simulink model "PICController"  (R2022a)
settings: Solver=VariableStepAuto  StartTime=0.0  StopTime=1  RelTol=1e-3
settings Model: Creator=Jagadeesh  LastModifiedBy=Jagadeesh

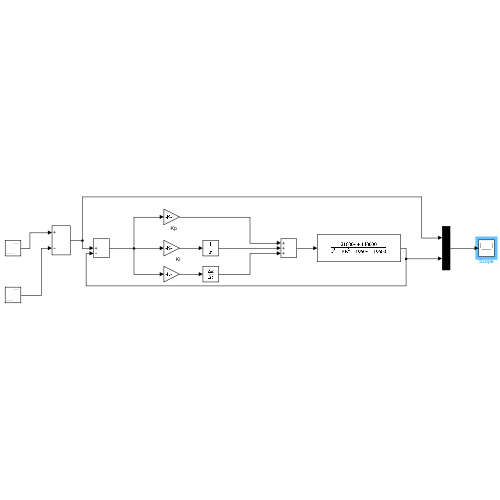
[thumbnail: Simulink's stored preview of the top-level diagram]
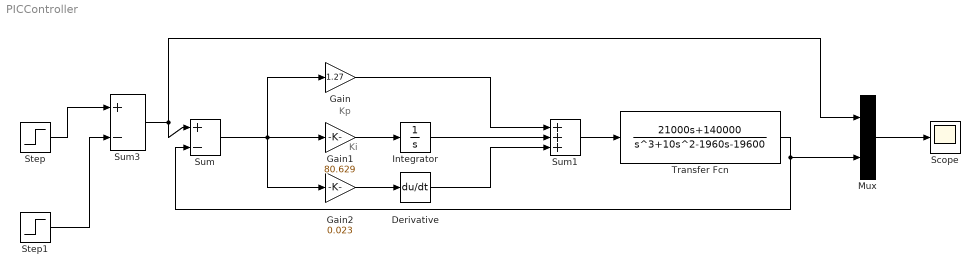
== system PICController ==
  note: Ki
  note: Kp
  Derivative : Derivative
  Gain : Gain  Gain=1.27
  Gain1 : Gain  Gain=80.629
  Gain2 : Gain  Gain=0.023
  Integrator : Integrator
  Mux : Mux  Inputs=2
  Scope : Scope
  Step : Step  Time=0  After=0.5  SampleTime=0
  Step1 : Step  Time=0.5  After=0.3  SampleTime=0
  Sum : Sum  Inputs=|+-
  Sum1 : Sum  Inputs=+++
  Sum3 : Sum  Inputs=+-
  Transfer Fcn : TransferFcn  Numerator=[21000 140000]  Denominator=[1 10 -1960 -19600]
  wires:
  Gain/1 -> Sum1/1
  Gain1/1 -> Integrator/1
  Derivative/1 -> Sum1/3
  Integrator/1 -> Sum1/2
  Transfer Fcn/1 -> Sum/2, Mux/2
  Sum/1 -> Gain/1, Gain2/1, Gain1/1
  Mux/1 -> Scope/1
  Sum1/1 -> Transfer Fcn/1
  Gain2/1 -> Derivative/1
  Step1/1 -> Sum3/2
  Step/1 -> Sum3/1
  Sum3/1 -> Mux/1, Sum/1
